simulink model "rti1401_program_controls_2018_test"  (R2017b)
settings: Solver=ode1  StartTime=0.0  StopTime=Inf  FixedStep=0.001  RelTol=1e-3  EnableMultiTasking=on
PreLoadFcn:
  | dataCar
  | load_vars
  | structAero
  | structEstimPar
  | structSensors
  | structSettings
PostLoadFcn:
  | , if any(exist('dsrtsu_mdlpostloadfcn', 'file') == [2, 3, 6]), try dsrtsu_mdlpostloadfcn('Execute', bdroot); catch fprintf('Error in PostLoadFcn (dsrtsu_mdlpostloadfcn) for model "%s":\n %s\n', bdroot, lasterr); end, end,
InitFcn:
  | dataCar
  | load_vars
  | structAero
  | structEstimPar
  | structSensors
  | structSettings
StartFcn:
  | dataCar
  | load_vars
  | structAero
  | structEstimPar
  | structSensors
  | structSettings
values from neighbouring files (symbols this model uses):
  Throttle_limits = [0.15, 0.90, 0.16, 0.92]    [load_vars.m]
undefined symbols (not defined in the file or in its folder): car, sensors
libraries: rtican x44, hdlsllib x32, simulink x8, rti1401lib_II_base x1
(part 2 of 11)

== system rti1401_program_controls_2018_test/Setup ==
  CAN_TYPE1_TX_M1_C1 : rtican/RTICAN Transmit (TX)   Reserved1=[]  Reserved2=[]  Reserved3=[]  Reserved4=[]  SfcnMessage=[]  Msg_Struct=[]  BoardTypeNo=[]  BoardNo=[]  ChannelNo=[]  Parameters=[]  DialogFcn=[]  UnitName=[]  Revision=[]  UnitValues=[]  DSProperties=struct('RTI',struct('Version',uint32(5),'BlockType',struct('isSLSource',uint8(1),'isSLSink',uint8(1),'isHWSource',uint8(0),'isHWSink',uint8(0),'isSetup',uint8(0),'isInline',uint8(1),'isNonInline',uint8(0),'isInterrupt',uint8(0),'isChannelwise',uint8(0)),'IOBoardType','RTICAN','UnitType','MESSAGE','Identifier','TX','DialogType','MSVC','BlockSet','RTICAN','SlaveProcessor','CAN'))  RTIBlockInterface=struct('InputPortsWidth',int32([1 1 1 1 1 1 1 1]),'InputPortsActive',[1 1 1 1 1 1 1 1],'InputPortsName',{{'Mux','dataByte1','dataByte2','dataByte3','dataByte4','dataByte5','dataByte6','dataByte7'}},'InputPortsDataType',{{'SS_UINT8','SS_UINT8','SS_UINT8','SS_UINT8','SS_UINT8','SS_UINT8','SS_UINT8','SS_UINT8'}},'OutputPortsWidth',int32(0),'OutputPortsActive',0,'OutputPortsName',{{''}},'DialogFcn','rtican_message_interface_gui','BlockDisplay',{{'','center'}},'IconTransparency','on','InitLevel',3,'BlockName',struct('Token',{{'CAN_TYPE','_TX_M','_C'}},'BlockParam',{{'BoardTypeNo','BoardNo','ChannelNo'}}),'SampleTime',{{-1}},'TriggerPort',{{'none'}},'EnablePort',{{'none'}})  RTIBlockParameters=struct('BoardTypeNo',{{1,'OFF',[]}},'BoardNo',{{1,'ON',[1 16]}},'ChannelNo',{{1,'ON',[1 2]}},'Parameters',{{struct('DataFileSupport',struct('DataFileSelectedMaster',0,'DataFileSelectedLocal',0,'DataFileName',['<no datafile support>|'],'DataFileDate','','SelectedFile',['<no file selected>']),'Options',struct('StatusSelected',0,'TimeSelected',0,'DeltaTimeSelected',0,'DelayTimeSelected',0,'DelayTimeTXCommandSelected',0,'EncodeSetUnusedBitsToOne',0,'EnableMsgLoopback',0,'TriggerPort',struct('Selected',0,'TriggerType',0),'EnablePortSelected',0,'SignalOnPortnameSelected',1,'UserCoding',struct('Selected',0,'InterfaceFile','UserEncodingFile','FcnName','UserEncodeFcn','InportSelected',0,'InportWidth',1,'OutportSelected',0,'OutportWidth',1),'TerminationMsg',struct('Selected',0,'Byte0_7','0'),'InitialMsg',struct('Selected',0,'Byte0_7','0')),'Message',struct('MsgOnBlocknameSelected',0,'MsgName','IVT_Msg_Command','MsgIdFormat',0,'MsgId',1041,'MsgLength',8,'NumSignals',8,'SampleTime',-1,'StartTime',struct('Selected',0,'Value',0),'AutoRepeatTime',struct('Selected',0,'Value',0.1),'Timeout',struct('Selected',0,'Value',0.1),'DelayTime',struct('Selected',0,'Value',0.1),'Signal',struct('SgnName',{'Mux','dataByte1','dataByte2','dataByte3','dataByte4','dataByte5','dataByte6','dataByte7'},'SgnStartBit',{0,8,16,24,32,40,48,56},'SgnLength',{8,8,8,8,8,8,8,8},'SgnType',{0,0,0,0,0,0,0,0},'ModeValue',{-1,-1,-1,-1,-1,-1,-1,-1},'DataType',{0,0,0,0,0,0,0,0},'ByteLayout',{1,1,1,1,1,1,1,1},'Factor',{1,1,1,1,1,1,1,1},'Offset',{0,0,0,0,0,0,0,0},'SgnComment',{{''},{''},{''},{''},{''},{''},{''},{''}},'SgnUnit',{'','','','','','','',''},'Min',{0,0,0,0,0,0,0,0},'Max',{255,255,255,255,255,255,255,255},'SLDataType',{'SS_UINT8','SS_UINT8','SS_UINT8','SS_UINT8','SS_UINT8','SS_UINT8','SS_UINT8','SS_UINT8'}),'MsgIdNumFormat',1,'MsgComment',{{''}}),'Version',1.2,'general',struct('isFromLib',0)),'OFF',[]}},'GroupId',{{struct('Group',{{'RTICAN'}},'No',1,'Behavior',{{'NAMECHANGE'}},'BlockType',{{'SINK'}},'NameChangeFlag',0),'OFF',[]}},'SFcnRTICANMessage',{{struct('MsgType','TX','SFcnPortType','Scalar','MsgName','IVT_Msg_Command','MsgIdFormat','STD','MsgId',1041,'MsgLength',8,'NumSignals',8,'SampleTime',-1,'StartTime',struct('Selected','no','Value',0),'AutoRepeatTime',struct('Selected','no','Value',0.1),'Timeout',struct('Selected','no','Value',0.1),'Signal',struct('SgnName',{'Mux','dataByte1','dataByte2','dataByte3','dataByte4','dataByte5','dataByte6','dataByte7'},'SgnStartBit',{0,8,16,24,32,40,48,56},'SgnLength',{8,8,8,8,8,8,8,8},'SgnType',{'standard','standard','standard','standard','standard','standard','standard','standard'},'ModeValue',{-1,-1,-1,-1,-1,-1,-1,-1},'DataType',{['unsigned int'],['unsigned int'],['unsigned int'],['unsigned int'],['unsigned int'],['unsigned int'],['unsigned int'],['unsigned int']},'ByteLayout',{['big endian'],['big endian'],['big endian'],['big endian'],['big endian'],['big endian'],['big endian'],['big endian']},'Factor',{1,1,1,1,1,1,1,1},'Offset',{0,0,0,0,0,0,0,0},'SLDataType',{'SS_UINT8','SS_UINT8','SS_UINT8','SS_UINT8','SS_UINT8','SS_UINT8','SS_UINT8','SS_UINT8'}),'StatusSelected','no','TimeSelected','no','DeltaTimeSelected','no','DelayTimeSelected','no','DelayTimeTXCommandSelected','no','EncodeSetUnusedBitsToOne','no','EnableMsgLoopback','no','TriggerPort',struct('Selected','no','TriggerType',0),'EnablePortSelected','no','UserCoding',struct('Selected','no','InterfaceFile','UserEncodingFile','FcnName','UserEncodeFcn','InportSelected','no','InportWidth',1,'OutportSelected','no','OutportWidth',1),'TerminationMsg',struct('Selected','no','Byte0','0x00','Byte1','0x00','Byte2','0x00','Byte3','0x00','Byte4','0x00','Byte5','0x00','Byte6','0x00','Byte7','0x00'),'InitialMsg',struct('Selected','no','Byte0','0x00','Byte1','0x00','Byte2','0x00','Byte3','0x00','Byte4','0x00','Byte5','0x00','Byte6','0x00','Byte7','0x00'),'BoardType','DS1','BoardNo',1,'ControllerNo',1),'OFF',[]}},'TLCFileName',{{'rtican_tx_message','OFF',[]}})  RTISFcnParameters=struct('SFcnRTICANMessage','struct','TLCFileName','char')  RTIBlockParaDefault=struct('BoardTypeNo',4302,'BoardNo',1,'ChannelNo',1,'Parameters',struct('DataFileSupport',struct('DataFileSelectedMaster',0,'DataFileSelectedLocal',0,'DataFileName','','DataFileDate','','SelectedFile',['<no file selected>']),'Options',struct('StatusSelected',1,'TimeSelected',1,'DeltaTimeSelected',1,'DelayTimeSelected',1,'DelayTimeTXCommandSelected',0,'EncodeSetUnusedBitsToOne',0,'EnableMsgLoopback',0,'TriggerPort',struct('Selected',0,'TriggerType','rising'),'EnablePortSelected',0,'SignalOnPortnameSelected',1,'UserCoding',struct('Selected',0,'InterfaceFile','UserEncodingFile','FcnName','UserEncodeFcn','InportSelected',0,'InportWidth',1,'OutportSelected',0,'OutportWidth',1),'TerminationMsg',struct('Selected',0,'Byte0_7','0'),'InitialMsg',struct('Selected',0,'Byte0_7','0')),'Message',struct('MsgOnBlocknameSelected',0,'MsgName',['TX Message'],'MsgIdFormat',0,'MsgId',100,'MsgLength',8,'NumSignals',1,'SampleTime',-1,'StartTime',struct('Selected',0,'Value',0),'AutoRepeatTime',struct('Selected',0,'Value',0.1),'Timeout',struct('Selected',0,'Value',0.1),'DelayTime',struct('Selected',0,'Value',0.1),'Signal',struct('SgnName',['TX signal'],'SgnStartBit',0,'SgnLength',8,'SgnType',0,'ModeValue',-1,'DataType',0,'SLDataType','SS_DOUBLE','ByteLayout',0,'Factor',1,'Offset',0,'Min',0,'Max',255,'SgnComment',{{}},'SgnUnit',''),'MsgIdNumFormat',0,'MsgComment',{{''}}),'Version',1.2,'general',struct('isFromLib',1)),'GroupId',struct('Group',{{'RTICAN'}},'No',1,'Behavior',{{'NAMECHANGE'}},'BlockType',{{'SINK'}},'NameChangeFlag',0),'SFcnRTICANMessage',struct('MsgType','TX','MsgName',['TX Message'],'MsgIdFormat','STD','MsgId',100,'MsgLength',2,'NumSignals',1,'SampleTime',-1,'StartTime',struct('Selected','no','Value',0),'AutoRepeatTime',struct('Selected','no','Value',0.1),'Timeout',struct('Selected','no','Value',0.1),'DelayTime',struct('Selected','no','Value',0.1),'Signal',struct('SgnName',['TX signal'],'SgnStartBit',0,'SgnLength',8,'SgnType','standard','ModeValue',-1,'DataType',['unsigned int'],'ByteLayout',['little endian'],'SLDataType','SS_DOUBLE','Factor',1,'Offset',0),'StatusSelected','yes','TimeSelected','yes','DeltaTimeSelected','yes','DelayTimeSelected','yes','EnablePortSelected','no','EnableMsgLoopback','no','DelayTimeTXCommandSelected','no','EncodeSetUnusedBitsToOne','no','UserCoding',struct('Selected','no','InterfaceFile','UserDecodingFile','FcnName','UserDecodeFcn','InportSelected','no','InportWidth',1,'OutportSelected','no','OutportWidth',1),'TerminationMsg',struct('Selected','no','Byte0','0x00','Byte1','0x00','Byte2','0x00','Byte3','0x00','Byte4','0x00','Byte5','0x00','Byte6','0x00','Byte7','0x00'),'InitialMsg',struct('Selected','no','Byte0','0x00','Byte1','0x00','Byte2','0x00','Byte3','0x00','Byte4','0x00','Byte5','0x00','Byte6','0x00','Byte7','0x00'),'TriggerPort',struct('Selected','no','TriggerType','rising'),'BoardType','DS4302','BoardNo',1,'ControllerNo',1,'SFcnPortType','Scalar'),'TLCFileName','rtican_tx_message')
      settings: AttributesFormatString=Group Id: RTICAN1\n
  Delay : Delay  DelayLength=1
  MATLAB Function : MATLAB Function  TreatAsAtomicUnit=on
  SETUP_CAN_DMC_FRONT : rtican/RTICAN CONTROLLER SETUP   Reserved1=[]  Reserved2=[]  Reserved3=[]  Reserved4=[]  AcceptanceMask=[]  ArbitrationField=[]  Parameters=[]  SFcnRTICANSettings=[]  MS_Struct=[]  BoardTypeNo=[]  BoardNo=[]  ChannelNo=[]  DialogFcn=[]  UnitName=[]  Revision=[]  UnitValues=[]  DSProperties=struct('RTI',struct('Version',uint32(12),'BlockType',struct('isSLSource',uint8(0),'isSLSink',uint8(0),'isHWSource',uint8(0),'isHWSink',uint8(0),'isSetup',uint8(1),'isInline',uint8(1),'isNonInline',uint8(0),'isInterrupt',uint8(0),'isChannelwise',uint8(0)),'IOBoardType','RTICAN','UnitType','NON_MESSAGE','Identifier','MASTER','DialogType','ML','BlockSet','RTICAN','SlaveProcessor','CAN'))  RTIBlockInterface=struct('InputPortsWidth',int32(0),'InputPortsActive',0,'OutputPortsWidth',int32(0),'OutputPortsActive',0,'DialogFcn','rtican_master_setup_gui','BlockDisplay',{{['CAN CONTROLLER\n SETUP'],'center'}},'IconTransparency','on','InitLevel',3,'IWork',{{{'',uint32(2)}}},'BlockName',struct('Token',{{'CAN_TYPE','_SETUP_M','_C'}},'BlockParam',{{'BoardTypeNo','BoardNo','ChannelNo'}}),'ParameterTunableNames',{{}})  RTIBlockParameters="struct('BoardTypeNo',{{1,'OFF',[]}},'BoardNo',{{1,'ON',[1 16]}},'ChannelNo',{{2,'ON',[1 2]}},'AcceptanceMask',{{0,'OFF',[]}},'ArbitrationField',{{0,'OFF',[]}},'Parameters',{{struct('Config',struct('Baudrate',1000,'SampleMode',1,'UsedParamSet',1,'validSettings',1,'isBTRvalues',0,'Advanced',struct('Baudrate',{500,500,500},'Frequency',{24000000,36000000,64000000},'Settings',{struct('SMPL',0,'BRP',0,'NBT',24,'TSEG1',15,'TSEG2',6,'SJW',3,'SP',70),struct('SMPL',0,'BRP',1,'NBT',18,'TSEG1',14,'TSEG2',1,'SJW',1,'SP',88),struct('SMPL',0,'BRP',3,'NBT',16,'TSEG1',12,'TSEG2',1,'SJW',1,'SP',87)},'BTR0',{192,65,67},'BTR1',{111,30,28})),'configType',1,'Options',struct('DataFileSelected',0,'DataFileName',{{['<no datafile support>']}},'DataFileDate',{{''}},'InterfaceFcn','rtican_dbc_file_parser','InterfaceFcnFileName','','LabelConfigType','volatile','AcceptanceMaskSelected',0,'MsgDataType','SgnSpecification','NumType','hex','MaskType','STD','AcceptanceMask',0,'ArbitrationField',0,'UseMultipleMessageAccess',0),'RxReceiveStdOptions',struct('RxServiceStdEnabled',0,'RxServiceStdMsgIdent',1000,'RxServiceStdIdentNumType',1,'RxServiceStdIdentMask',0,'RxServiceStdMaskNumType',1,'RxServiceStdQueueSize',64),'RxReceiveXtdOptions',struct('RxServiceXtdEnabled',0,'RxServiceXtdMsgIdent',1001,'RxServiceXtdIdentNumType',1,'RxServiceXtdIdentMask',0,'RxServiceXtdMaskNumType',1,'RxServiceXtdQueueSize',64),'PartialNetworkingOptions',struct('switchedon',0,'format',1,'idmask',['    XXXXX XXXXXXXX XXXXXXXX XXXXXXXX'],'idcode','0','idfilter','0','datamaskused',0,'datalength',1,'datamask','0x0000000000000000','partialnetworkenable',0),'general',struct('Termination_common',1,'Termination_C252',1,'BusConfigurationRegister',0,'Transceiver','ISO11898','isFromLib',0)),'OFF',[]}},'CCPParameters',{{struct('CRO',struct('Format','STD','NumFormat','hex','Id',1639),'DTO',struct('Format','STD','NumFormat','hex','Id',2017),'StationAdr',struct('NumFormat','hex','Value',57),'StationId',struct('Value',['dSPACE CCP Service']),'Enabled',0),'OFF',[]}},'XCPParameters',{{struct('MASTER',struct('Format','STD','NumFormat','hex','Id',256),'SLAVE',struct('Format','STD','NumFormat','hex','Id',510),'Enabled',0,'PIDTransmissionEnabled',0),'OFF',[]}},'GroupId',{{struct('Group',{{'RTICAN'}},'No',2,'Behavior',{{'EVER'}},'BlockType',{{'SOURCE'}},'NameChangeFlag',1),'OFF',[]}},'SFcnRTICANSettings',{{struct('Baudrate',1000,'configType',1,'AdvancedConfig',struct('Frequency',{},'BTR0',{},'BTR1',{}),'UsedParamSet',1,'STDMaskSelected','no','XTDMaskSelected','no','BoardType','DS1','BoardNo',1,'ControllerNo',2,'Transceiver','ISO11898','BusConfigRegister',0,'TerminationRes',120,'UseMultipleMessageAccess','no','STDRXSrvcUsed','no','STDRXSrvcMsgId',1000,'STDRXSrvcMsgMask',0,'STDRXSrvcQueueSize',64,'XTDRXSrvcUsed','no','XTDRXSrvcMsgId',1001,'XTDRXSrvcQueueSize',64,'XTDRXSrvcMsgMask',0,'PN_IsPNTransciever',0,'PN_IsPNEnabled',0,'PN_MsgFormat',1,'PN_idcode',0,'PN_idmask',2047,'PN_datamaskused',0,'PN_datalength',0,'PN_datamask',['0xFF, 0xFF, 0xFF, 0xFF, 0xFF, 0xFF, 0xFF, 0xFF']),'OFF',[]}},'SFcnRTICCPSettings',{{struct('CRO',struct('Format','STD','NumFormat','hex','Id',1639),'DTO',struct('Format','STD','NumFormat','hex','Id',2017),'StationAdr',struct('NumFormat','hex','Value',57),'StationId',struct('Value',['dSPACE CCP Service']),'Enabled',0),'OFF',[]}},'SFcnRTIXCPSettings',{{struct('MASTER',struct('Format','STD','NumFormat','hex','Id',256),'SLAVE',struct('Format','STD','NumFormat','hex','Id',510),'Enabled',0,'PIDTransmissionEnabled',0),'OFF',[]}},'TLCFileName',{{'rtican_master_setup','OFF',[]}})"  RTISFcnParameters=struct('SFcnRTICANSettings','struct','SFcnRTICCPSettings','struct','SFcnRTIXCPSettings','struct','AcceptanceMask','int32','ArbitrationField','int32','TLCFileName','char')  RTIBlockParaDefault="struct('BoardTypeNo',4302,'BoardNo',1,'ChannelNo',1,'AcceptanceMask',0,'ArbitrationField',0,'Parameters',struct('Config',struct('Baudrate',500,'SampleMode',1,'UsedParamSet',1,'validSettings',1,'isBTRvalues',0,'Advanced',struct('Frequency',16000000,'BTR0',64,'BTR1',28,'Settings',struct('SMPL',0,'BRP',0,'NBT',16,'TSEG1',12,'TSEG2',1,'SJW',1,'SP',87))),'configType',1,'Options',struct('DataFileSelected',0,'DataFileName',{{['<no datafile support>']}},'DataFileDate',{{''}},'InterfaceFcn','rtican_dbc_file_parser','InterfaceFcnFileName','','LabelConfigType','volatile','AcceptanceMaskSelected',0,'MsgDataType','AllwaysDouble','NumType','hex','MaskType','STD','AcceptanceMask',0,'ArbitrationField',0,'UseMultipleMessageAccess',0),'RxReceiveStdOptions',struct('RxServiceStdEnabled',0,'RxServiceStdMsgIdent',1000,'RxServiceStdIdentNumType',1,'RxServiceStdIdentMask',0,'RxServiceStdMaskNumType',1,'RxServiceStdQueueSize',64),'RxReceiveXtdOptions',struct('RxServiceXtdEnabled',0,'RxServiceXtdMsgIdent',1001,'RxServiceXtdIdentNumType',1,'RxServiceXtdIdentMask',0,'RxServiceXtdMaskNumType',1,'RxServiceXtdQueueSize',64),'PartialNetworkingOptions',struct('switchedon',0,'format',1,'idmask',['    XXXXX XXXXXXXX XXXXXXXX XXXXXXXX'],'idcode','0','idfilter','0','datamaskused',0,'datalength',1,'datamask','0x0000000000000000','partialnetworkenable',0),'general',struct('Termination_common',1,'Termination_C252',1,'BusConfigurationRegister',0,'Transceiver','ISO11898','isFromLib',1)),'CCPParameters',struct('CRO',struct('Format','STD','NumFormat','hex','Id',1639),'DTO',struct('Format','STD','NumFormat','hex','Id',2017),'StationAdr',struct('NumFormat','hex','Value',57),'StationId',struct('Value',['dSPACE CCP Service']),'Enabled',0),'XCPParameters',struct('MASTER',struct('Format','STD','NumFormat','hex','Id',256),'SLAVE',struct('Format','STD','NumFormat','hex','Id',510),'Enabled',0,'PIDTransmissionEnabled',0),'GroupId',struct('Group',{{'RTICAN'}},'No',1,'Behavior',{{'EVER'}},'BlockType',{{'SOURCE'}},'NameChangeFlag',1),'SFcnRTICANSettings',struct('Baudrate',500,'configType',1,'AdvandedConfig',struct('Frequency',16000000,'BTR0','0x40','BTR1','0x1C'),'UsedParamSet',1,'STDMaskSelected','no','XTDMaskSelected','no','BoardType','DS4302','BoardNo',1,'ControllerNo',1,'Transceiver','ISO11898','BusConfigRegister',0,'TerminationRes',120,'UseMultipleMessageAccess','no','STDRXSrvcUsed','no','STDRXSrvcMsgId',1000,'STDRXSrvcMsgMask',0,'STDRXSrvcQueueSize',64,'XTDRXSrvcUsed','no','XTDRXSrvcMsgId',1001,'XTDRXSrvcQueueSize',64,'XTDRXSrvcMsgMask',0),'SFcnRTICCPSettings',struct('CRO',struct('Format','STD','NumFormat','hex','Id',1639),'DTO',struct('Format','STD','NumFormat','hex','Id',2017),'StationAdr',struct('NumFormat','hex','Value',57),'StationId',struct('Value',['dSPACE CCP Service']),'Enabled',0),'SFcnRTIXCPSettings',struct('MASTER',struct('Format','STD','NumFormat','hex','Id',256),'SLAVE',struct('Format','STD','NumFormat','hex','Id',510),'Enabled',0,'PIDTransmissionEnabled',0),'TLCFileName','rtican_master_setup')"
      settings: AttributesFormatString=Group Id: RTICAN2\n
  SETUP_CAN_DMC_REAR : rtican/RTICAN CONTROLLER SETUP   Reserved1=[]  Reserved2=[]  Reserved3=[]  Reserved4=[]  AcceptanceMask=[]  ArbitrationField=[]  Parameters=[]  SFcnRTICANSettings=[]  MS_Struct=[]  BoardTypeNo=[]  BoardNo=[]  ChannelNo=[]  DialogFcn=[]  UnitName=[]  Revision=[]  UnitValues=[]  DSProperties=struct('RTI',struct('Version',uint32(12),'BlockType',struct('isSLSource',uint8(0),'isSLSink',uint8(0),'isHWSource',uint8(0),'isHWSink',uint8(0),'isSetup',uint8(1),'isInline',uint8(1),'isNonInline',uint8(0),'isInterrupt',uint8(0),'isChannelwise',uint8(0)),'IOBoardType','RTICAN','UnitType','NON_MESSAGE','Identifier','MASTER','DialogType','ML','BlockSet','RTICAN','SlaveProcessor','CAN'))  RTIBlockInterface=struct('InputPortsWidth',int32(0),'InputPortsActive',0,'OutputPortsWidth',int32(0),'OutputPortsActive',0,'DialogFcn','rtican_master_setup_gui','BlockDisplay',{{['CAN CONTROLLER\n SETUP'],'center'}},'IconTransparency','on','InitLevel',3,'IWork',{{{'',uint32(2)}}},'BlockName',struct('Token',{{'CAN_TYPE','_SETUP_M','_C'}},'BlockParam',{{'BoardTypeNo','BoardNo','ChannelNo'}}),'ParameterTunableNames',{{}})  RTIBlockParameters="struct('BoardTypeNo',{{1,'OFF',[]}},'BoardNo',{{2,'ON',[1 16]}},'ChannelNo',{{1,'ON',[1 2]}},'AcceptanceMask',{{0,'OFF',[]}},'ArbitrationField',{{0,'OFF',[]}},'Parameters',{{struct('Config',struct('Baudrate',1000,'SampleMode',1,'UsedParamSet',1,'validSettings',1,'isBTRvalues',0,'Advanced',struct('Baudrate',{500,500,500},'Frequency',{24000000,36000000,64000000},'Settings',{struct('SMPL',0,'BRP',0,'NBT',24,'TSEG1',15,'TSEG2',6,'SJW',3,'SP',70),struct('SMPL',0,'BRP',1,'NBT',18,'TSEG1',14,'TSEG2',1,'SJW',1,'SP',88),struct('SMPL',0,'BRP',3,'NBT',16,'TSEG1',12,'TSEG2',1,'SJW',1,'SP',87)},'BTR0',{192,65,67},'BTR1',{111,30,28})),'configType',1,'Options',struct('DataFileSelected',0,'DataFileName',{{['<no datafile support>']}},'DataFileDate',{{''}},'InterfaceFcn','rtican_dbc_file_parser','InterfaceFcnFileName','','LabelConfigType','volatile','AcceptanceMaskSelected',0,'MsgDataType','SgnSpecification','NumType','hex','MaskType','STD','AcceptanceMask',0,'ArbitrationField',0,'UseMultipleMessageAccess',0),'RxReceiveStdOptions',struct('RxServiceStdEnabled',0,'RxServiceStdMsgIdent',1000,'RxServiceStdIdentNumType',1,'RxServiceStdIdentMask',0,'RxServiceStdMaskNumType',1,'RxServiceStdQueueSize',64),'RxReceiveXtdOptions',struct('RxServiceXtdEnabled',0,'RxServiceXtdMsgIdent',1001,'RxServiceXtdIdentNumType',1,'RxServiceXtdIdentMask',0,'RxServiceXtdMaskNumType',1,'RxServiceXtdQueueSize',64),'PartialNetworkingOptions',struct('switchedon',0,'format',1,'idmask',['    XXXXX XXXXXXXX XXXXXXXX XXXXXXXX'],'idcode','0','idfilter','0','datamaskused',0,'datalength',1,'datamask','0x0000000000000000','partialnetworkenable',0),'general',struct('Termination_common',1,'Termination_C252',1,'BusConfigurationRegister',0,'Transceiver','ISO11898','isFromLib',0)),'OFF',[]}},'CCPParameters',{{struct('CRO',struct('Format','STD','NumFormat','hex','Id',1639),'DTO',struct('Format','STD','NumFormat','hex','Id',2017),'StationAdr',struct('NumFormat','hex','Value',57),'StationId',struct('Value',['dSPACE CCP Service']),'Enabled',0),'OFF',[]}},'XCPParameters',{{struct('MASTER',struct('Format','STD','NumFormat','hex','Id',256),'SLAVE',struct('Format','STD','NumFormat','hex','Id',510),'Enabled',0,'PIDTransmissionEnabled',0),'OFF',[]}},'GroupId',{{struct('Group',{{'RTICAN'}},'No',3,'Behavior',{{'EVER'}},'BlockType',{{'SOURCE'}},'NameChangeFlag',1),'OFF',[]}},'SFcnRTICANSettings',{{struct('Baudrate',1000,'configType',1,'AdvancedConfig',struct('Frequency',{},'BTR0',{},'BTR1',{}),'UsedParamSet',1,'STDMaskSelected','no','XTDMaskSelected','no','BoardType','DS1','BoardNo',2,'ControllerNo',1,'Transceiver','ISO11898','BusConfigRegister',0,'TerminationRes',120,'UseMultipleMessageAccess','no','STDRXSrvcUsed','no','STDRXSrvcMsgId',1000,'STDRXSrvcMsgMask',0,'STDRXSrvcQueueSize',64,'XTDRXSrvcUsed','no','XTDRXSrvcMsgId',1001,'XTDRXSrvcQueueSize',64,'XTDRXSrvcMsgMask',0,'PN_IsPNTransciever',0,'PN_IsPNEnabled',0,'PN_MsgFormat',1,'PN_idcode',0,'PN_idmask',2047,'PN_datamaskused',0,'PN_datalength',0,'PN_datamask',['0xFF, 0xFF, 0xFF, 0xFF, 0xFF, 0xFF, 0xFF, 0xFF']),'OFF',[]}},'SFcnRTICCPSettings',{{struct('CRO',struct('Format','STD','NumFormat','hex','Id',1639),'DTO',struct('Format','STD','NumFormat','hex','Id',2017),'StationAdr',struct('NumFormat','hex','Value',57),'StationId',struct('Value',['dSPACE CCP Service']),'Enabled',0),'OFF',[]}},'SFcnRTIXCPSettings',{{struct('MASTER',struct('Format','STD','NumFormat','hex','Id',256),'SLAVE',struct('Format','STD','NumFormat','hex','Id',510),'Enabled',0,'PIDTransmissionEnabled',0),'OFF',[]}},'TLCFileName',{{'rtican_master_setup','OFF',[]}})"  RTISFcnParameters=struct('SFcnRTICANSettings','struct','SFcnRTICCPSettings','struct','SFcnRTIXCPSettings','struct','AcceptanceMask','int32','ArbitrationField','int32','TLCFileName','char')  RTIBlockParaDefault="struct('BoardTypeNo',4302,'BoardNo',1,'ChannelNo',1,'AcceptanceMask',0,'ArbitrationField',0,'Parameters',struct('Config',struct('Baudrate',500,'SampleMode',1,'UsedParamSet',1,'validSettings',1,'isBTRvalues',0,'Advanced',struct('Frequency',16000000,'BTR0',64,'BTR1',28,'Settings',struct('SMPL',0,'BRP',0,'NBT',16,'TSEG1',12,'TSEG2',1,'SJW',1,'SP',87))),'configType',1,'Options',struct('DataFileSelected',0,'DataFileName',{{['<no datafile support>']}},'DataFileDate',{{''}},'InterfaceFcn','rtican_dbc_file_parser','InterfaceFcnFileName','','LabelConfigType','volatile','AcceptanceMaskSelected',0,'MsgDataType','AllwaysDouble','NumType','hex','MaskType','STD','AcceptanceMask',0,'ArbitrationField',0,'UseMultipleMessageAccess',0),'RxReceiveStdOptions',struct('RxServiceStdEnabled',0,'RxServiceStdMsgIdent',1000,'RxServiceStdIdentNumType',1,'RxServiceStdIdentMask',0,'RxServiceStdMaskNumType',1,'RxServiceStdQueueSize',64),'RxReceiveXtdOptions',struct('RxServiceXtdEnabled',0,'RxServiceXtdMsgIdent',1001,'RxServiceXtdIdentNumType',1,'RxServiceXtdIdentMask',0,'RxServiceXtdMaskNumType',1,'RxServiceXtdQueueSize',64),'PartialNetworkingOptions',struct('switchedon',0,'format',1,'idmask',['    XXXXX XXXXXXXX XXXXXXXX XXXXXXXX'],'idcode','0','idfilter','0','datamaskused',0,'datalength',1,'datamask','0x0000000000000000','partialnetworkenable',0),'general',struct('Termination_common',1,'Termination_C252',1,'BusConfigurationRegister',0,'Transceiver','ISO11898','isFromLib',1)),'CCPParameters',struct('CRO',struct('Format','STD','NumFormat','hex','Id',1639),'DTO',struct('Format','STD','NumFormat','hex','Id',2017),'StationAdr',struct('NumFormat','hex','Value',57),'StationId',struct('Value',['dSPACE CCP Service']),'Enabled',0),'XCPParameters',struct('MASTER',struct('Format','STD','NumFormat','hex','Id',256),'SLAVE',struct('Format','STD','NumFormat','hex','Id',510),'Enabled',0,'PIDTransmissionEnabled',0),'GroupId',struct('Group',{{'RTICAN'}},'No',1,'Behavior',{{'EVER'}},'BlockType',{{'SOURCE'}},'NameChangeFlag',1),'SFcnRTICANSettings',struct('Baudrate',500,'configType',1,'AdvandedConfig',struct('Frequency',16000000,'BTR0','0x40','BTR1','0x1C'),'UsedParamSet',1,'STDMaskSelected','no','XTDMaskSelected','no','BoardType','DS4302','BoardNo',1,'ControllerNo',1,'Transceiver','ISO11898','BusConfigRegister',0,'TerminationRes',120,'UseMultipleMessageAccess','no','STDRXSrvcUsed','no','STDRXSrvcMsgId',1000,'STDRXSrvcMsgMask',0,'STDRXSrvcQueueSize',64,'XTDRXSrvcUsed','no','XTDRXSrvcMsgId',1001,'XTDRXSrvcQueueSize',64,'XTDRXSrvcMsgMask',0),'SFcnRTICCPSettings',struct('CRO',struct('Format','STD','NumFormat','hex','Id',1639),'DTO',struct('Format','STD','NumFormat','hex','Id',2017),'StationAdr',struct('NumFormat','hex','Value',57),'StationId',struct('Value',['dSPACE CCP Service']),'Enabled',0),'SFcnRTIXCPSettings',struct('MASTER',struct('Format','STD','NumFormat','hex','Id',256),'SLAVE',struct('Format','STD','NumFormat','hex','Id',510),'Enabled',0,'PIDTransmissionEnabled',0),'TLCFileName','rtican_master_setup')"
      settings: AttributesFormatString=Group Id: RTICAN3\n
  SETUP_CAN_ENERGY : rtican/RTICAN CONTROLLER SETUP   Reserved1=[]  Reserved2=[]  Reserved3=[]  Reserved4=[]  AcceptanceMask=[]  ArbitrationField=[]  Parameters=[]  SFcnRTICANSettings=[]  MS_Struct=[]  BoardTypeNo=[]  BoardNo=[]  ChannelNo=[]  DialogFcn=[]  UnitName=[]  Revision=[]  UnitValues=[]  DSProperties=struct('RTI',struct('Version',uint32(12),'BlockType',struct('isSLSource',uint8(0),'isSLSink',uint8(0),'isHWSource',uint8(0),'isHWSink',uint8(0),'isSetup',uint8(1),'isInline',uint8(1),'isNonInline',uint8(0),'isInterrupt',uint8(0),'isChannelwise',uint8(0)),'IOBoardType','RTICAN','UnitType','NON_MESSAGE','Identifier','MASTER','DialogType','ML','BlockSet','RTICAN','SlaveProcessor','CAN'))  RTIBlockInterface=struct('InputPortsWidth',int32(0),'InputPortsActive',0,'OutputPortsWidth',int32(0),'OutputPortsActive',0,'DialogFcn','rtican_master_setup_gui','BlockDisplay',{{['CAN CONTROLLER\n SETUP'],'center'}},'IconTransparency','on','InitLevel',3,'IWork',{{{'',uint32(2)}}},'BlockName',struct('Token',{{'CAN_TYPE','_SETUP_M','_C'}},'BlockParam',{{'BoardTypeNo','BoardNo','ChannelNo'}}),'ParameterTunableNames',{{}})  RTIBlockParameters="struct('BoardTypeNo',{{1,'OFF',[]}},'BoardNo',{{2,'ON',[1 16]}},'ChannelNo',{{2,'ON',[1 2]}},'AcceptanceMask',{{0,'OFF',[]}},'ArbitrationField',{{0,'OFF',[]}},'Parameters',{{struct('Config',struct('Baudrate',500,'SampleMode',1,'UsedParamSet',1,'validSettings',1,'isBTRvalues',0,'Advanced',struct('Baudrate',{500,500,500},'Frequency',{24000000,36000000,64000000},'Settings',{struct('SMPL',0,'BRP',0,'NBT',24,'TSEG1',15,'TSEG2',6,'SJW',3,'SP',70),struct('SMPL',0,'BRP',1,'NBT',18,'TSEG1',14,'TSEG2',1,'SJW',1,'SP',88),struct('SMPL',0,'BRP',3,'NBT',16,'TSEG1',12,'TSEG2',1,'SJW',1,'SP',87)},'BTR0',{192,65,67},'BTR1',{111,30,28})),'configType',1,'Options',struct('DataFileSelected',0,'DataFileName',{{['<no datafile support>']}},'DataFileDate',{{''}},'InterfaceFcn','rtican_dbc_file_parser','InterfaceFcnFileName','','LabelConfigType','volatile','AcceptanceMaskSelected',0,'MsgDataType','SgnSpecification','NumType','hex','MaskType','STD','AcceptanceMask',0,'ArbitrationField',0,'UseMultipleMessageAccess',0),'RxReceiveStdOptions',struct('RxServiceStdEnabled',0,'RxServiceStdMsgIdent',1000,'RxServiceStdIdentNumType',1,'RxServiceStdIdentMask',0,'RxServiceStdMaskNumType',1,'RxServiceStdQueueSize',64),'RxReceiveXtdOptions',struct('RxServiceXtdEnabled',0,'RxServiceXtdMsgIdent',1001,'RxServiceXtdIdentNumType',1,'RxServiceXtdIdentMask',0,'RxServiceXtdMaskNumType',1,'RxServiceXtdQueueSize',64),'PartialNetworkingOptions',struct('switchedon',0,'format',1,'idmask',['    XXXXX XXXXXXXX XXXXXXXX XXXXXXXX'],'idcode','0','idfilter','0','datamaskused',0,'datalength',1,'datamask','0x0000000000000000','partialnetworkenable',0),'general',struct('Termination_common',1,'Termination_C252',1,'BusConfigurationRegister',0,'Transceiver','ISO11898','isFromLib',0)),'OFF',[]}},'CCPParameters',{{struct('CRO',struct('Format','STD','NumFormat','hex','Id',1639),'DTO',struct('Format','STD','NumFormat','hex','Id',2017),'StationAdr',struct('NumFormat','hex','Value',57),'StationId',struct('Value',['dSPACE CCP Service']),'Enabled',0),'OFF',[]}},'XCPParameters',{{struct('MASTER',struct('Format','STD','NumFormat','hex','Id',256),'SLAVE',struct('Format','STD','NumFormat','hex','Id',510),'Enabled',0,'PIDTransmissionEnabled',0),'OFF',[]}},'GroupId',{{struct('Group',{{'RTICAN'}},'No',4,'Behavior',{{'EVER'}},'BlockType',{{'SOURCE'}},'NameChangeFlag',1),'OFF',[]}},'SFcnRTICANSettings',{{struct('Baudrate',500,'configType',1,'AdvancedConfig',struct('Frequency',{},'BTR0',{},'BTR1',{}),'UsedParamSet',1,'STDMaskSelected','no','XTDMaskSelected','no','BoardType','DS1','BoardNo',2,'ControllerNo',2,'Transceiver','ISO11898','BusConfigRegister',0,'TerminationRes',120,'UseMultipleMessageAccess','no','STDRXSrvcUsed','no','STDRXSrvcMsgId',1000,'STDRXSrvcMsgMask',0,'STDRXSrvcQueueSize',64,'XTDRXSrvcUsed','no','XTDRXSrvcMsgId',1001,'XTDRXSrvcQueueSize',64,'XTDRXSrvcMsgMask',0,'PN_IsPNTransciever',0,'PN_IsPNEnabled',0,'PN_MsgFormat',1,'PN_idcode',0,'PN_idmask',2047,'PN_datamaskused',0,'PN_datalength',0,'PN_datamask',['0xFF, 0xFF, 0xFF, 0xFF, 0xFF, 0xFF, 0xFF, 0xFF']),'OFF',[]}},'SFcnRTICCPSettings',{{struct('CRO',struct('Format','STD','NumFormat','hex','Id',1639),'DTO',struct('Format','STD','NumFormat','hex','Id',2017),'StationAdr',struct('NumFormat','hex','Value',57),'StationId',struct('Value',['dSPACE CCP Service']),'Enabled',0),'OFF',[]}},'SFcnRTIXCPSettings',{{struct('MASTER',struct('Format','STD','NumFormat','hex','Id',256),'SLAVE',struct('Format','STD','NumFormat','hex','Id',510),'Enabled',0,'PIDTransmissionEnabled',0),'OFF',[]}},'TLCFileName',{{'rtican_master_setup','OFF',[]}})"  RTISFcnParameters=struct('SFcnRTICANSettings','struct','SFcnRTICCPSettings','struct','SFcnRTIXCPSettings','struct','AcceptanceMask','int32','ArbitrationField','int32','TLCFileName','char')  RTIBlockParaDefault="struct('BoardTypeNo',4302,'BoardNo',1,'ChannelNo',1,'AcceptanceMask',0,'ArbitrationField',0,'Parameters',struct('Config',struct('Baudrate',500,'SampleMode',1,'UsedParamSet',1,'validSettings',1,'isBTRvalues',0,'Advanced',struct('Frequency',16000000,'BTR0',64,'BTR1',28,'Settings',struct('SMPL',0,'BRP',0,'NBT',16,'TSEG1',12,'TSEG2',1,'SJW',1,'SP',87))),'configType',1,'Options',struct('DataFileSelected',0,'DataFileName',{{['<no datafile support>']}},'DataFileDate',{{''}},'InterfaceFcn','rtican_dbc_file_parser','InterfaceFcnFileName','','LabelConfigType','volatile','AcceptanceMaskSelected',0,'MsgDataType','AllwaysDouble','NumType','hex','MaskType','STD','AcceptanceMask',0,'ArbitrationField',0,'UseMultipleMessageAccess',0),'RxReceiveStdOptions',struct('RxServiceStdEnabled',0,'RxServiceStdMsgIdent',1000,'RxServiceStdIdentNumType',1,'RxServiceStdIdentMask',0,'RxServiceStdMaskNumType',1,'RxServiceStdQueueSize',64),'RxReceiveXtdOptions',struct('RxServiceXtdEnabled',0,'RxServiceXtdMsgIdent',1001,'RxServiceXtdIdentNumType',1,'RxServiceXtdIdentMask',0,'RxServiceXtdMaskNumType',1,'RxServiceXtdQueueSize',64),'PartialNetworkingOptions',struct('switchedon',0,'format',1,'idmask',['    XXXXX XXXXXXXX XXXXXXXX XXXXXXXX'],'idcode','0','idfilter','0','datamaskused',0,'datalength',1,'datamask','0x0000000000000000','partialnetworkenable',0),'general',struct('Termination_common',1,'Termination_C252',1,'BusConfigurationRegister',0,'Transceiver','ISO11898','isFromLib',1)),'CCPParameters',struct('CRO',struct('Format','STD','NumFormat','hex','Id',1639),'DTO',struct('Format','STD','NumFormat','hex','Id',2017),'StationAdr',struct('NumFormat','hex','Value',57),'StationId',struct('Value',['dSPACE CCP Service']),'Enabled',0),'XCPParameters',struct('MASTER',struct('Format','STD','NumFormat','hex','Id',256),'SLAVE',struct('Format','STD','NumFormat','hex','Id',510),'Enabled',0,'PIDTransmissionEnabled',0),'GroupId',struct('Group',{{'RTICAN'}},'No',1,'Behavior',{{'EVER'}},'BlockType',{{'SOURCE'}},'NameChangeFlag',1),'SFcnRTICANSettings',struct('Baudrate',500,'configType',1,'AdvandedConfig',struct('Frequency',16000000,'BTR0','0x40','BTR1','0x1C'),'UsedParamSet',1,'STDMaskSelected','no','XTDMaskSelected','no','BoardType','DS4302','BoardNo',1,'ControllerNo',1,'Transceiver','ISO11898','BusConfigRegister',0,'TerminationRes',120,'UseMultipleMessageAccess','no','STDRXSrvcUsed','no','STDRXSrvcMsgId',1000,'STDRXSrvcMsgMask',0,'STDRXSrvcQueueSize',64,'XTDRXSrvcUsed','no','XTDRXSrvcMsgId',1001,'XTDRXSrvcQueueSize',64,'XTDRXSrvcMsgMask',0),'SFcnRTICCPSettings',struct('CRO',struct('Format','STD','NumFormat','hex','Id',1639),'DTO',struct('Format','STD','NumFormat','hex','Id',2017),'StationAdr',struct('NumFormat','hex','Value',57),'StationId',struct('Value',['dSPACE CCP Service']),'Enabled',0),'SFcnRTIXCPSettings',struct('MASTER',struct('Format','STD','NumFormat','hex','Id',256),'SLAVE',struct('Format','STD','NumFormat','hex','Id',510),'Enabled',0,'PIDTransmissionEnabled',0),'TLCFileName','rtican_master_setup')"
      settings: AttributesFormatString=Group Id: RTICAN4\n
  SETUP_CAN_FRONT : rtican/RTICAN CONTROLLER SETUP   Reserved1=[]  Reserved2=[]  Reserved3=[]  Reserved4=[]  AcceptanceMask=[]  ArbitrationField=[]  Parameters=[]  SFcnRTICANSettings=[]  MS_Struct=[]  BoardTypeNo=[]  BoardNo=[]  ChannelNo=[]  DialogFcn=[]  UnitName=[]  Revision=[]  UnitValues=[]  DSProperties=struct('RTI',struct('Version',uint32(12),'BlockType',struct('isSLSource',uint8(0),'isSLSink',uint8(0),'isHWSource',uint8(0),'isHWSink',uint8(0),'isSetup',uint8(1),'isInline',uint8(1),'isNonInline',uint8(0),'isInterrupt',uint8(0),'isChannelwise',uint8(0)),'IOBoardType','RTICAN','UnitType','NON_MESSAGE','Identifier','MASTER','DialogType','ML','BlockSet','RTICAN','SlaveProcessor','CAN'))  RTIBlockInterface=struct('InputPortsWidth',int32(0),'InputPortsActive',0,'OutputPortsWidth',int32(0),'OutputPortsActive',0,'DialogFcn','rtican_master_setup_gui','BlockDisplay',{{['CAN CONTROLLER\n SETUP'],'center'}},'IconTransparency','on','InitLevel',3,'IWork',{{{'',uint32(2)}}},'BlockName',struct('Token',{{'CAN_TYPE','_SETUP_M','_C'}},'BlockParam',{{'BoardTypeNo','BoardNo','ChannelNo'}}),'ParameterTunableNames',{{}})  RTIBlockParameters="struct('BoardTypeNo',{{1,'OFF',[]}},'BoardNo',{{1,'ON',[1 16]}},'ChannelNo',{{1,'ON',[1 2]}},'AcceptanceMask',{{0,'OFF',[]}},'ArbitrationField',{{0,'OFF',[]}},'Parameters',{{struct('Config',struct('Baudrate',500,'SampleMode',1,'UsedParamSet',1,'validSettings',1,'isBTRvalues',0,'Advanced',struct('Baudrate',{500,500,500},'Frequency',{24000000,36000000,64000000},'Settings',{struct('SMPL',0,'BRP',0,'NBT',24,'TSEG1',15,'TSEG2',6,'SJW',3,'SP',70),struct('SMPL',0,'BRP',1,'NBT',18,'TSEG1',14,'TSEG2',1,'SJW',1,'SP',88),struct('SMPL',0,'BRP',3,'NBT',16,'TSEG1',12,'TSEG2',1,'SJW',1,'SP',87)},'BTR0',{192,65,67},'BTR1',{111,30,28})),'configType',1,'Options',struct('DataFileSelected',0,'DataFileName',{{['<no datafile support>']}},'DataFileDate',{{''}},'InterfaceFcn','rtican_dbc_file_parser','InterfaceFcnFileName','','LabelConfigType','volatile','AcceptanceMaskSelected',0,'MsgDataType','SgnSpecification','NumType','hex','MaskType','STD','AcceptanceMask',0,'ArbitrationField',0,'UseMultipleMessageAccess',0),'RxReceiveStdOptions',struct('RxServiceStdEnabled',0,'RxServiceStdMsgIdent',1000,'RxServiceStdIdentNumType',1,'RxServiceStdIdentMask',0,'RxServiceStdMaskNumType',1,'RxServiceStdQueueSize',64),'RxReceiveXtdOptions',struct('RxServiceXtdEnabled',0,'RxServiceXtdMsgIdent',1001,'RxServiceXtdIdentNumType',1,'RxServiceXtdIdentMask',0,'RxServiceXtdMaskNumType',1,'RxServiceXtdQueueSize',64),'PartialNetworkingOptions',struct('switchedon',0,'format',1,'idmask',['    XXXXX XXXXXXXX XXXXXXXX XXXXXXXX'],'idcode','0','idfilter','0','datamaskused',0,'datalength',1,'datamask','0x0000000000000000','partialnetworkenable',0),'general',struct('Termination_common',1,'Termination_C252',1,'BusConfigurationRegister',0,'Transceiver','ISO11898','isFromLib',0)),'OFF',[]}},'CCPParameters',{{struct('CRO',struct('Format','STD','NumFormat','hex','Id',1639),'DTO',struct('Format','STD','NumFormat','hex','Id',2017),'StationAdr',struct('NumFormat','hex','Value',57),'StationId',struct('Value',['dSPACE CCP Service']),'Enabled',0),'OFF',[]}},'XCPParameters',{{struct('MASTER',struct('Format','STD','NumFormat','hex','Id',256),'SLAVE',struct('Format','STD','NumFormat','hex','Id',510),'Enabled',0,'PIDTransmissionEnabled',0),'OFF',[]}},'GroupId',{{struct('Group',{{'RTICAN'}},'No',1,'Behavior',{{'EVER'}},'BlockType',{{'SOURCE'}},'NameChangeFlag',1),'OFF',[]}},'SFcnRTICANSettings',{{struct('Baudrate',500,'configType',1,'AdvancedConfig',struct('Frequency',{},'BTR0',{},'BTR1',{}),'UsedParamSet',1,'STDMaskSelected','no','XTDMaskSelected','no','BoardType','DS1','BoardNo',1,'ControllerNo',1,'Transceiver','ISO11898','BusConfigRegister',0,'TerminationRes',120,'UseMultipleMessageAccess','no','STDRXSrvcUsed','no','STDRXSrvcMsgId',1000,'STDRXSrvcMsgMask',0,'STDRXSrvcQueueSize',64,'XTDRXSrvcUsed','no','XTDRXSrvcMsgId',1001,'XTDRXSrvcQueueSize',64,'XTDRXSrvcMsgMask',0,'PN_IsPNTransciever',0,'PN_IsPNEnabled',0,'PN_MsgFormat',1,'PN_idcode',0,'PN_idmask',2047,'PN_datamaskused',0,'PN_datalength',0,'PN_datamask',['0xFF, 0xFF, 0xFF, 0xFF, 0xFF, 0xFF, 0xFF, 0xFF']),'OFF',[]}},'SFcnRTICCPSettings',{{struct('CRO',struct('Format','STD','NumFormat','hex','Id',1639),'DTO',struct('Format','STD','NumFormat','hex','Id',2017),'StationAdr',struct('NumFormat','hex','Value',57),'StationId',struct('Value',['dSPACE CCP Service']),'Enabled',0),'OFF',[]}},'SFcnRTIXCPSettings',{{struct('MASTER',struct('Format','STD','NumFormat','hex','Id',256),'SLAVE',struct('Format','STD','NumFormat','hex','Id',510),'Enabled',0,'PIDTransmissionEnabled',0),'OFF',[]}},'TLCFileName',{{'rtican_master_setup','OFF',[]}})"  RTISFcnParameters=struct('SFcnRTICANSettings','struct','SFcnRTICCPSettings','struct','SFcnRTIXCPSettings','struct','AcceptanceMask','int32','ArbitrationField','int32','TLCFileName','char')  RTIBlockParaDefault="struct('BoardTypeNo',4302,'BoardNo',1,'ChannelNo',1,'AcceptanceMask',0,'ArbitrationField',0,'Parameters',struct('Config',struct('Baudrate',500,'SampleMode',1,'UsedParamSet',1,'validSettings',1,'isBTRvalues',0,'Advanced',struct('Frequency',16000000,'BTR0',64,'BTR1',28,'Settings',struct('SMPL',0,'BRP',0,'NBT',16,'TSEG1',12,'TSEG2',1,'SJW',1,'SP',87))),'configType',1,'Options',struct('DataFileSelected',0,'DataFileName',{{['<no datafile support>']}},'DataFileDate',{{''}},'InterfaceFcn','rtican_dbc_file_parser','InterfaceFcnFileName','','LabelConfigType','volatile','AcceptanceMaskSelected',0,'MsgDataType','AllwaysDouble','NumType','hex','MaskType','STD','AcceptanceMask',0,'ArbitrationField',0,'UseMultipleMessageAccess',0),'RxReceiveStdOptions',struct('RxServiceStdEnabled',0,'RxServiceStdMsgIdent',1000,'RxServiceStdIdentNumType',1,'RxServiceStdIdentMask',0,'RxServiceStdMaskNumType',1,'RxServiceStdQueueSize',64),'RxReceiveXtdOptions',struct('RxServiceXtdEnabled',0,'RxServiceXtdMsgIdent',1001,'RxServiceXtdIdentNumType',1,'RxServiceXtdIdentMask',0,'RxServiceXtdMaskNumType',1,'RxServiceXtdQueueSize',64),'PartialNetworkingOptions',struct('switchedon',0,'format',1,'idmask',['    XXXXX XXXXXXXX XXXXXXXX XXXXXXXX'],'idcode','0','idfilter','0','datamaskused',0,'datalength',1,'datamask','0x0000000000000000','partialnetworkenable',0),'general',struct('Termination_common',1,'Termination_C252',1,'BusConfigurationRegister',0,'Transceiver','ISO11898','isFromLib',1)),'CCPParameters',struct('CRO',struct('Format','STD','NumFormat','hex','Id',1639),'DTO',struct('Format','STD','NumFormat','hex','Id',2017),'StationAdr',struct('NumFormat','hex','Value',57),'StationId',struct('Value',['dSPACE CCP Service']),'Enabled',0),'XCPParameters',struct('MASTER',struct('Format','STD','NumFormat','hex','Id',256),'SLAVE',struct('Format','STD','NumFormat','hex','Id',510),'Enabled',0,'PIDTransmissionEnabled',0),'GroupId',struct('Group',{{'RTICAN'}},'No',1,'Behavior',{{'EVER'}},'BlockType',{{'SOURCE'}},'NameChangeFlag',1),'SFcnRTICANSettings',struct('Baudrate',500,'configType',1,'AdvandedConfig',struct('Frequency',16000000,'BTR0','0x40','BTR1','0x1C'),'UsedParamSet',1,'STDMaskSelected','no','XTDMaskSelected','no','BoardType','DS4302','BoardNo',1,'ControllerNo',1,'Transceiver','ISO11898','BusConfigRegister',0,'TerminationRes',120,'UseMultipleMessageAccess','no','STDRXSrvcUsed','no','STDRXSrvcMsgId',1000,'STDRXSrvcMsgMask',0,'STDRXSrvcQueueSize',64,'XTDRXSrvcUsed','no','XTDRXSrvcMsgId',1001,'XTDRXSrvcQueueSize',64,'XTDRXSrvcMsgMask',0),'SFcnRTICCPSettings',struct('CRO',struct('Format','STD','NumFormat','hex','Id',1639),'DTO',struct('Format','STD','NumFormat','hex','Id',2017),'StationAdr',struct('NumFormat','hex','Value',57),'StationId',struct('Value',['dSPACE CCP Service']),'Enabled',0),'SFcnRTIXCPSettings',struct('MASTER',struct('Format','STD','NumFormat','hex','Id',256),'SLAVE',struct('Format','STD','NumFormat','hex','Id',510),'Enabled',0,'PIDTransmissionEnabled',0),'TLCFileName','rtican_master_setup')"
      settings: AttributesFormatString=Group Id: RTICAN1\n
  SETUP_CAN_REAR : rtican/RTICAN CONTROLLER SETUP   Reserved1=[]  Reserved2=[]  Reserved3=[]  Reserved4=[]  AcceptanceMask=[]  ArbitrationField=[]  Parameters=[]  SFcnRTICANSettings=[]  MS_Struct=[]  BoardTypeNo=[]  BoardNo=[]  ChannelNo=[]  DialogFcn=[]  UnitName=[]  Revision=[]  UnitValues=[]  DSProperties=struct('RTI',struct('Version',uint32(12),'BlockType',struct('isSLSource',uint8(0),'isSLSink',uint8(0),'isHWSource',uint8(0),'isHWSink',uint8(0),'isSetup',uint8(1),'isInline',uint8(1),'isNonInline',uint8(0),'isInterrupt',uint8(0),'isChannelwise',uint8(0)),'IOBoardType','RTICAN','UnitType','NON_MESSAGE','Identifier','MASTER','DialogType','ML','BlockSet','RTICAN','SlaveProcessor','CAN'))  RTIBlockInterface=struct('InputPortsWidth',int32(0),'InputPortsActive',0,'OutputPortsWidth',int32(0),'OutputPortsActive',0,'DialogFcn','rtican_master_setup_gui','BlockDisplay',{{['CAN CONTROLLER\n SETUP'],'center'}},'IconTransparency','on','InitLevel',3,'IWork',{{{'',uint32(2)}}},'BlockName',struct('Token',{{'CAN_TYPE','_SETUP_M','_C'}},'BlockParam',{{'BoardTypeNo','BoardNo','ChannelNo'}}),'ParameterTunableNames',{{}})  RTIBlockParameters="struct('BoardTypeNo',{{1,'OFF',[]}},'BoardNo',{{3,'ON',[1 16]}},'ChannelNo',{{1,'ON',[1 2]}},'AcceptanceMask',{{0,'OFF',[]}},'ArbitrationField',{{0,'OFF',[]}},'Parameters',{{struct('Config',struct('Baudrate',500,'SampleMode',1,'UsedParamSet',1,'validSettings',1,'isBTRvalues',0,'Advanced',struct('Baudrate',{500,500,500},'Frequency',{24000000,36000000,64000000},'Settings',{struct('SMPL',0,'BRP',0,'NBT',24,'TSEG1',15,'TSEG2',6,'SJW',3,'SP',70),struct('SMPL',0,'BRP',1,'NBT',18,'TSEG1',14,'TSEG2',1,'SJW',1,'SP',88),struct('SMPL',0,'BRP',3,'NBT',16,'TSEG1',12,'TSEG2',1,'SJW',1,'SP',87)},'BTR0',{192,65,67},'BTR1',{111,30,28})),'configType',1,'Options',struct('DataFileSelected',0,'DataFileName',{{['<no datafile support>']}},'DataFileDate',{{''}},'InterfaceFcn','rtican_dbc_file_parser','InterfaceFcnFileName','','LabelConfigType','volatile','AcceptanceMaskSelected',0,'MsgDataType','SgnSpecification','NumType','hex','MaskType','STD','AcceptanceMask',0,'ArbitrationField',0,'UseMultipleMessageAccess',0),'RxReceiveStdOptions',struct('RxServiceStdEnabled',0,'RxServiceStdMsgIdent',1000,'RxServiceStdIdentNumType',1,'RxServiceStdIdentMask',0,'RxServiceStdMaskNumType',1,'RxServiceStdQueueSize',64),'RxReceiveXtdOptions',struct('RxServiceXtdEnabled',0,'RxServiceXtdMsgIdent',1001,'RxServiceXtdIdentNumType',1,'RxServiceXtdIdentMask',0,'RxServiceXtdMaskNumType',1,'RxServiceXtdQueueSize',64),'PartialNetworkingOptions',struct('switchedon',0,'format',1,'idmask',['    XXXXX XXXXXXXX XXXXXXXX XXXXXXXX'],'idcode','0','idfilter','0','datamaskused',0,'datalength',1,'datamask','0x0000000000000000','partialnetworkenable',0),'general',struct('Termination_common',1,'Termination_C252',1,'BusConfigurationRegister',0,'Transceiver','ISO11898','isFromLib',0)),'OFF',[]}},'CCPParameters',{{struct('CRO',struct('Format','STD','NumFormat','hex','Id',1639),'DTO',struct('Format','STD','NumFormat','hex','Id',2017),'StationAdr',struct('NumFormat','hex','Value',57),'StationId',struct('Value',['dSPACE CCP Service']),'Enabled',0),'OFF',[]}},'XCPParameters',{{struct('MASTER',struct('Format','STD','NumFormat','hex','Id',256),'SLAVE',struct('Format','STD','NumFormat','hex','Id',510),'Enabled',0,'PIDTransmissionEnabled',0),'OFF',[]}},'GroupId',{{struct('Group',{{'RTICAN'}},'No',5,'Behavior',{{'EVER'}},'BlockType',{{'SOURCE'}},'NameChangeFlag',1),'OFF',[]}},'SFcnRTICANSettings',{{struct('Baudrate',500,'configType',1,'AdvancedConfig',struct('Frequency',{},'BTR0',{},'BTR1',{}),'UsedParamSet',1,'STDMaskSelected','no','XTDMaskSelected','no','BoardType','DS1','BoardNo',3,'ControllerNo',1,'Transceiver','ISO11898','BusConfigRegister',0,'TerminationRes',120,'UseMultipleMessageAccess','no','STDRXSrvcUsed','no','STDRXSrvcMsgId',1000,'STDRXSrvcMsgMask',0,'STDRXSrvcQueueSize',64,'XTDRXSrvcUsed','no','XTDRXSrvcMsgId',1001,'XTDRXSrvcQueueSize',64,'XTDRXSrvcMsgMask',0,'PN_IsPNTransciever',0,'PN_IsPNEnabled',0,'PN_MsgFormat',1,'PN_idcode',0,'PN_idmask',2047,'PN_datamaskused',0,'PN_datalength',0,'PN_datamask',['0xFF, 0xFF, 0xFF, 0xFF, 0xFF, 0xFF, 0xFF, 0xFF']),'OFF',[]}},'SFcnRTICCPSettings',{{struct('CRO',struct('Format','STD','NumFormat','hex','Id',1639),'DTO',struct('Format','STD','NumFormat','hex','Id',2017),'StationAdr',struct('NumFormat','hex','Value',57),'StationId',struct('Value',['dSPACE CCP Service']),'Enabled',0),'OFF',[]}},'SFcnRTIXCPSettings',{{struct('MASTER',struct('Format','STD','NumFormat','hex','Id',256),'SLAVE',struct('Format','STD','NumFormat','hex','Id',510),'Enabled',0,'PIDTransmissionEnabled',0),'OFF',[]}},'TLCFileName',{{'rtican_master_setup','OFF',[]}})"  RTISFcnParameters=struct('SFcnRTICANSettings','struct','SFcnRTICCPSettings','struct','SFcnRTIXCPSettings','struct','AcceptanceMask','int32','ArbitrationField','int32','TLCFileName','char')  RTIBlockParaDefault="struct('BoardTypeNo',4302,'BoardNo',1,'ChannelNo',1,'AcceptanceMask',0,'ArbitrationField',0,'Parameters',struct('Config',struct('Baudrate',500,'SampleMode',1,'UsedParamSet',1,'validSettings',1,'isBTRvalues',0,'Advanced',struct('Frequency',16000000,'BTR0',64,'BTR1',28,'Settings',struct('SMPL',0,'BRP',0,'NBT',16,'TSEG1',12,'TSEG2',1,'SJW',1,'SP',87))),'configType',1,'Options',struct('DataFileSelected',0,'DataFileName',{{['<no datafile support>']}},'DataFileDate',{{''}},'InterfaceFcn','rtican_dbc_file_parser','InterfaceFcnFileName','','LabelConfigType','volatile','AcceptanceMaskSelected',0,'MsgDataType','AllwaysDouble','NumType','hex','MaskType','STD','AcceptanceMask',0,'ArbitrationField',0,'UseMultipleMessageAccess',0),'RxReceiveStdOptions',struct('RxServiceStdEnabled',0,'RxServiceStdMsgIdent',1000,'RxServiceStdIdentNumType',1,'RxServiceStdIdentMask',0,'RxServiceStdMaskNumType',1,'RxServiceStdQueueSize',64),'RxReceiveXtdOptions',struct('RxServiceXtdEnabled',0,'RxServiceXtdMsgIdent',1001,'RxServiceXtdIdentNumType',1,'RxServiceXtdIdentMask',0,'RxServiceXtdMaskNumType',1,'RxServiceXtdQueueSize',64),'PartialNetworkingOptions',struct('switchedon',0,'format',1,'idmask',['    XXXXX XXXXXXXX XXXXXXXX XXXXXXXX'],'idcode','0','idfilter','0','datamaskused',0,'datalength',1,'datamask','0x0000000000000000','partialnetworkenable',0),'general',struct('Termination_common',1,'Termination_C252',1,'BusConfigurationRegister',0,'Transceiver','ISO11898','isFromLib',1)),'CCPParameters',struct('CRO',struct('Format','STD','NumFormat','hex','Id',1639),'DTO',struct('Format','STD','NumFormat','hex','Id',2017),'StationAdr',struct('NumFormat','hex','Value',57),'StationId',struct('Value',['dSPACE CCP Service']),'Enabled',0),'XCPParameters',struct('MASTER',struct('Format','STD','NumFormat','hex','Id',256),'SLAVE',struct('Format','STD','NumFormat','hex','Id',510),'Enabled',0,'PIDTransmissionEnabled',0),'GroupId',struct('Group',{{'RTICAN'}},'No',1,'Behavior',{{'EVER'}},'BlockType',{{'SOURCE'}},'NameChangeFlag',1),'SFcnRTICANSettings',struct('Baudrate',500,'configType',1,'AdvandedConfig',struct('Frequency',16000000,'BTR0','0x40','BTR1','0x1C'),'UsedParamSet',1,'STDMaskSelected','no','XTDMaskSelected','no','BoardType','DS4302','BoardNo',1,'ControllerNo',1,'Transceiver','ISO11898','BusConfigRegister',0,'TerminationRes',120,'UseMultipleMessageAccess','no','STDRXSrvcUsed','no','STDRXSrvcMsgId',1000,'STDRXSrvcMsgMask',0,'STDRXSrvcQueueSize',64,'XTDRXSrvcUsed','no','XTDRXSrvcMsgId',1001,'XTDRXSrvcQueueSize',64,'XTDRXSrvcMsgMask',0),'SFcnRTICCPSettings',struct('CRO',struct('Format','STD','NumFormat','hex','Id',1639),'DTO',struct('Format','STD','NumFormat','hex','Id',2017),'StationAdr',struct('NumFormat','hex','Value',57),'StationId',struct('Value',['dSPACE CCP Service']),'Enabled',0),'SFcnRTIXCPSettings',struct('MASTER',struct('Format','STD','NumFormat','hex','Id',256),'SLAVE',struct('Format','STD','NumFormat','hex','Id',510),'Enabled',0,'PIDTransmissionEnabled',0),'TLCFileName','rtican_master_setup')"
      settings: AttributesFormatString=Group Id: RTICAN5\n
  SETUP_CAN_YRS : rtican/RTICAN CONTROLLER SETUP   Reserved1=[]  Reserved2=[]  Reserved3=[]  Reserved4=[]  AcceptanceMask=[]  ArbitrationField=[]  Parameters=[]  SFcnRTICANSettings=[]  MS_Struct=[]  BoardTypeNo=[]  BoardNo=[]  ChannelNo=[]  DialogFcn=[]  UnitName=[]  Revision=[]  UnitValues=[]  DSProperties=struct('RTI',struct('Version',uint32(12),'BlockType',struct('isSLSource',uint8(0),'isSLSink',uint8(0),'isHWSource',uint8(0),'isHWSink',uint8(0),'isSetup',uint8(1),'isInline',uint8(1),'isNonInline',uint8(0),'isInterrupt',uint8(0),'isChannelwise',uint8(0)),'IOBoardType','RTICAN','UnitType','NON_MESSAGE','Identifier','MASTER','DialogType','ML','BlockSet','RTICAN','SlaveProcessor','CAN'))  RTIBlockInterface=struct('InputPortsWidth',int32(0),'InputPortsActive',0,'OutputPortsWidth',int32(0),'OutputPortsActive',0,'DialogFcn','rtican_master_setup_gui','BlockDisplay',{{['CAN CONTROLLER\n SETUP'],'center'}},'IconTransparency','on','InitLevel',3,'IWork',{{{'',uint32(2)}}},'BlockName',struct('Token',{{'CAN_TYPE','_SETUP_M','_C'}},'BlockParam',{{'BoardTypeNo','BoardNo','ChannelNo'}}),'ParameterTunableNames',{{}})  RTIBlockParameters="struct('BoardTypeNo',{{1,'OFF',[]}},'BoardNo',{{3,'ON',[1 16]}},'ChannelNo',{{2,'ON',[1 2]}},'AcceptanceMask',{{0,'OFF',[]}},'ArbitrationField',{{0,'OFF',[]}},'Parameters',{{struct('Config',struct('Baudrate',1000,'SampleMode',1,'UsedParamSet',1,'validSettings',1,'isBTRvalues',0,'Advanced',struct('Baudrate',{500,500,500},'Frequency',{24000000,36000000,64000000},'Settings',{struct('SMPL',0,'BRP',0,'NBT',24,'TSEG1',15,'TSEG2',6,'SJW',3,'SP',70),struct('SMPL',0,'BRP',1,'NBT',18,'TSEG1',14,'TSEG2',1,'SJW',1,'SP',88),struct('SMPL',0,'BRP',3,'NBT',16,'TSEG1',12,'TSEG2',1,'SJW',1,'SP',87)},'BTR0',{192,65,67},'BTR1',{111,30,28})),'configType',1,'Options',struct('DataFileSelected',0,'DataFileName',{{['<no datafile support>']}},'DataFileDate',{{''}},'InterfaceFcn','rtican_dbc_file_parser','InterfaceFcnFileName','','LabelConfigType','volatile','AcceptanceMaskSelected',0,'MsgDataType','SgnSpecification','NumType','hex','MaskType','STD','AcceptanceMask',0,'ArbitrationField',0,'UseMultipleMessageAccess',0),'RxReceiveStdOptions',struct('RxServiceStdEnabled',0,'RxServiceStdMsgIdent',1000,'RxServiceStdIdentNumType',1,'RxServiceStdIdentMask',0,'RxServiceStdMaskNumType',1,'RxServiceStdQueueSize',64),'RxReceiveXtdOptions',struct('RxServiceXtdEnabled',0,'RxServiceXtdMsgIdent',1001,'RxServiceXtdIdentNumType',1,'RxServiceXtdIdentMask',0,'RxServiceXtdMaskNumType',1,'RxServiceXtdQueueSize',64),'PartialNetworkingOptions',struct('switchedon',0,'format',1,'idmask',['    XXXXX XXXXXXXX XXXXXXXX XXXXXXXX'],'idcode','0','idfilter','0','datamaskused',0,'datalength',1,'datamask','0x0000000000000000','partialnetworkenable',0),'general',struct('Termination_common',1,'Termination_C252',1,'BusConfigurationRegister',0,'Transceiver','ISO11898','isFromLib',0)),'OFF',[]}},'CCPParameters',{{struct('CRO',struct('Format','STD','NumFormat','hex','Id',1639),'DTO',struct('Format','STD','NumFormat','hex','Id',2017),'StationAdr',struct('NumFormat','hex','Value',57),'StationId',struct('Value',['dSPACE CCP Service']),'Enabled',0),'OFF',[]}},'XCPParameters',{{struct('MASTER',struct('Format','STD','NumFormat','hex','Id',256),'SLAVE',struct('Format','STD','NumFormat','hex','Id',510),'Enabled',0,'PIDTransmissionEnabled',0),'OFF',[]}},'GroupId',{{struct('Group',{{'RTICAN'}},'No',6,'Behavior',{{'EVER'}},'BlockType',{{'SOURCE'}},'NameChangeFlag',1),'OFF',[]}},'SFcnRTICANSettings',{{struct('Baudrate',1000,'configType',1,'AdvancedConfig',struct('Frequency',{},'BTR0',{},'BTR1',{}),'UsedParamSet',1,'STDMaskSelected','no','XTDMaskSelected','no','BoardType','DS1','BoardNo',3,'ControllerNo',2,'Transceiver','ISO11898','BusConfigRegister',0,'TerminationRes',120,'UseMultipleMessageAccess','no','STDRXSrvcUsed','no','STDRXSrvcMsgId',1000,'STDRXSrvcMsgMask',0,'STDRXSrvcQueueSize',64,'XTDRXSrvcUsed','no','XTDRXSrvcMsgId',1001,'XTDRXSrvcQueueSize',64,'XTDRXSrvcMsgMask',0,'PN_IsPNTransciever',0,'PN_IsPNEnabled',0,'PN_MsgFormat',1,'PN_idcode',0,'PN_idmask',2047,'PN_datamaskused',0,'PN_datalength',0,'PN_datamask',['0xFF, 0xFF, 0xFF, 0xFF, 0xFF, 0xFF, 0xFF, 0xFF']),'OFF',[]}},'SFcnRTICCPSettings',{{struct('CRO',struct('Format','STD','NumFormat','hex','Id',1639),'DTO',struct('Format','STD','NumFormat','hex','Id',2017),'StationAdr',struct('NumFormat','hex','Value',57),'StationId',struct('Value',['dSPACE CCP Service']),'Enabled',0),'OFF',[]}},'SFcnRTIXCPSettings',{{struct('MASTER',struct('Format','STD','NumFormat','hex','Id',256),'SLAVE',struct('Format','STD','NumFormat','hex','Id',510),'Enabled',0,'PIDTransmissionEnabled',0),'OFF',[]}},'TLCFileName',{{'rtican_master_setup','OFF',[]}})"  RTISFcnParameters=struct('SFcnRTICANSettings','struct','SFcnRTICCPSettings','struct','SFcnRTIXCPSettings','struct','AcceptanceMask','int32','ArbitrationField','int32','TLCFileName','char')  RTIBlockParaDefault="struct('BoardTypeNo',4302,'BoardNo',1,'ChannelNo',1,'AcceptanceMask',0,'ArbitrationField',0,'Parameters',struct('Config',struct('Baudrate',500,'SampleMode',1,'UsedParamSet',1,'validSettings',1,'isBTRvalues',0,'Advanced',struct('Frequency',16000000,'BTR0',64,'BTR1',28,'Settings',struct('SMPL',0,'BRP',0,'NBT',16,'TSEG1',12,'TSEG2',1,'SJW',1,'SP',87))),'configType',1,'Options',struct('DataFileSelected',0,'DataFileName',{{['<no datafile support>']}},'DataFileDate',{{''}},'InterfaceFcn','rtican_dbc_file_parser','InterfaceFcnFileName','','LabelConfigType','volatile','AcceptanceMaskSelected',0,'MsgDataType','AllwaysDouble','NumType','hex','MaskType','STD','AcceptanceMask',0,'ArbitrationField',0,'UseMultipleMessageAccess',0),'RxReceiveStdOptions',struct('RxServiceStdEnabled',0,'RxServiceStdMsgIdent',1000,'RxServiceStdIdentNumType',1,'RxServiceStdIdentMask',0,'RxServiceStdMaskNumType',1,'RxServiceStdQueueSize',64),'RxReceiveXtdOptions',struct('RxServiceXtdEnabled',0,'RxServiceXtdMsgIdent',1001,'RxServiceXtdIdentNumType',1,'RxServiceXtdIdentMask',0,'RxServiceXtdMaskNumType',1,'RxServiceXtdQueueSize',64),'PartialNetworkingOptions',struct('switchedon',0,'format',1,'idmask',['    XXXXX XXXXXXXX XXXXXXXX XXXXXXXX'],'idcode','0','idfilter','0','datamaskused',0,'datalength',1,'datamask','0x0000000000000000','partialnetworkenable',0),'general',struct('Termination_common',1,'Termination_C252',1,'BusConfigurationRegister',0,'Transceiver','ISO11898','isFromLib',1)),'CCPParameters',struct('CRO',struct('Format','STD','NumFormat','hex','Id',1639),'DTO',struct('Format','STD','NumFormat','hex','Id',2017),'StationAdr',struct('NumFormat','hex','Value',57),'StationId',struct('Value',['dSPACE CCP Service']),'Enabled',0),'XCPParameters',struct('MASTER',struct('Format','STD','NumFormat','hex','Id',256),'SLAVE',struct('Format','STD','NumFormat','hex','Id',510),'Enabled',0,'PIDTransmissionEnabled',0),'GroupId',struct('Group',{{'RTICAN'}},'No',1,'Behavior',{{'EVER'}},'BlockType',{{'SOURCE'}},'NameChangeFlag',1),'SFcnRTICANSettings',struct('Baudrate',500,'configType',1,'AdvandedConfig',struct('Frequency',16000000,'BTR0','0x40','BTR1','0x1C'),'UsedParamSet',1,'STDMaskSelected','no','XTDMaskSelected','no','BoardType','DS4302','BoardNo',1,'ControllerNo',1,'Transceiver','ISO11898','BusConfigRegister',0,'TerminationRes',120,'UseMultipleMessageAccess','no','STDRXSrvcUsed','no','STDRXSrvcMsgId',1000,'STDRXSrvcMsgMask',0,'STDRXSrvcQueueSize',64,'XTDRXSrvcUsed','no','XTDRXSrvcMsgId',1001,'XTDRXSrvcQueueSize',64,'XTDRXSrvcMsgMask',0),'SFcnRTICCPSettings',struct('CRO',struct('Format','STD','NumFormat','hex','Id',1639),'DTO',struct('Format','STD','NumFormat','hex','Id',2017),'StationAdr',struct('NumFormat','hex','Value',57),'StationId',struct('Value',['dSPACE CCP Service']),'Enabled',0),'SFcnRTIXCPSettings',struct('MASTER',struct('Format','STD','NumFormat','hex','Id',256),'SLAVE',struct('Format','STD','NumFormat','hex','Id',510),'Enabled',0,'PIDTransmissionEnabled',0),'TLCFileName','rtican_master_setup')"
      settings: AttributesFormatString=Group Id: RTICAN6\n
  wires:
  MATLAB Function/9(progress) -> Delay/1
  MATLAB Function/1(messageByte0) -> CAN_TYPE1_TX_M1_C1/1
  MATLAB Function/2(messageByte1) -> CAN_TYPE1_TX_M1_C1/2
  MATLAB Function/3(messageByte2) -> CAN_TYPE1_TX_M1_C1/3
  MATLAB Function/4(messageByte3) -> CAN_TYPE1_TX_M1_C1/4
  MATLAB Function/5(messageByte4) -> CAN_TYPE1_TX_M1_C1/5
  MATLAB Function/6(messageByte5) -> CAN_TYPE1_TX_M1_C1/6
  MATLAB Function/7(messageByte6) -> CAN_TYPE1_TX_M1_C1/7
  MATLAB Function/8(messageByte7) -> CAN_TYPE1_TX_M1_C1/8
  Delay/1 -> MATLAB Function/1(initialProgress)
